simulink model "end_effector_position1"  (R2020a)
settings: Solver=VariableStepAuto  StartTime=0.0  StopTime=360  RelTol=1e-3
libraries: simulink x6
settings Model: Creator=Lord  LastModifiedBy=Lord

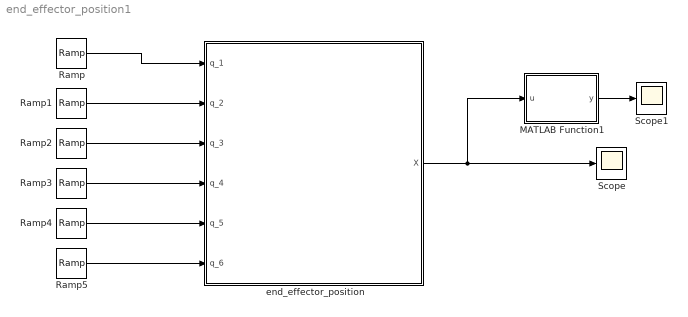
== system end_effector_position1 ==
  MATLAB Function1 : MATLAB Function  TreatAsAtomicUnit=on
  Ramp{,1..5} (6 alike) : simulink/Sources/Ramp  slope=1  start=0  InitialOutput=0
  Scope : Scope
  Scope1 : Scope
  end_effector_position : MATLAB Function  TreatAsAtomicUnit=on
  wires:
  end_effector_position/1(X) -> MATLAB Function1/1(u), Scope/1
  Ramp/1 -> end_effector_position/1(q_1)
  MATLAB Function1/1(y) -> Scope1/1
  Ramp5/1 -> end_effector_position/6(q_6)
  Ramp4/1 -> end_effector_position/5(q_5)
  Ramp3/1 -> end_effector_position/4(q_4)
  Ramp2/1 -> end_effector_position/3(q_3)
  Ramp1/1 -> end_effector_position/2(q_2)

== matlab function end_effector_position1/MATLAB Function1 ==
  data: u input; y output
function y = fcn(u)
t = 0:1:360;
xt1 = u(1)*t;
yt1 = u(2)*t;
zt1 = u(3)*t;
plot3(xt1,yt1,zt1)
y = u;

== matlab function end_effector_position1/end_effector_position ==
  data: q_1 input; X output; q_2 input; q_3 input; q_4 input; q_5 input; q_6 input
function X = end_effector_position(q_1,q_2,q_3,q_4,q_5,q_6)
%T= sym('a', [4,4,6]);
q=[q_1 q_2 q_3 q_4 q_5 q_6];
l0=2;
l1=2;
l2=2;
l3=2;
l4=2;
l5=2;
l6=2;
DH_Table=[q_1 l0 l1 90;q_2 0 l2 0;q_3+90 0 0 90;q_4 l3+l4 0 -90;q_5 0 0 90;q_6 l5+l6 0 0]; 
d=zeros(1,6);
a=zeros(1,6);
alpha=zeros(1,6);
T=cell(4);


for i=1:1:6
    for j=1:1:4
            if j==2
              d(i)=DH_Table(i,j);
            elseif j==1
              q(i)=DH_Table(i,j);
            elseif j==3
              a(i)=DH_Table(i,j);
            else    
              alpha(i)=DH_Table(i,j);
            end
    end
    B=transformation_func(q(i),d(i),a(i),alpha(i));
    T{i}=B;
end

T_EE=T{1}*T{2}*T{3}*T{4}*T{5}*T{6};
Xpos=T_EE(1,4);
Ypos=T_EE(2,4);
Zpos=T_EE(3,4);
X= [Xpos,Ypos,Zpos]; %position vector
end
